simulink model "CrossCorrelation_SimulinkModel"  (R2018b)
settings: Solver=VariableStepAuto  StartTime=0.0  StopTime=0.1  RelTol=1e-3
libraries: dspstat3 x1
settings Model: Creator=Jayef  LastModifiedBy=Jayef

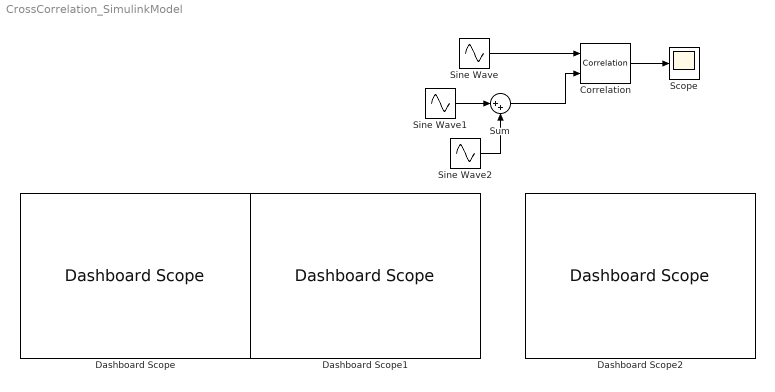
== system CrossCorrelation_SimulinkModel ==
  Correlation : dspstat3/Correlation  domain=Time  roundingMode=Floor  overflowMode=off  outputDataTypeStr=Inherit: Same as accumulator  outputMin=[]  outputMax=[]  outputLastDataTypeStr=Inherit: Same as accumulator
      settings: SourceProductName=DSP System Toolbox  SourceProductBaseCode=DS
  Dashboard Scope : DashboardScope  WebBlockId=4
  Dashboard Scope1 : DashboardScope  WebBlockId=9
  Dashboard Scope2 : DashboardScope  WebBlockId=10
  Scope : Scope
  Sine Wave : Sin  Frequency=2*3.14*50  SampleTime=1/1000
  Sine Wave1 : Sin  Frequency=2*3.14*50  SampleTime=1/1000
  Sine Wave2 : Sin  Amplitude=0.23  Frequency=2*3.14*70  SampleTime=1/1000
  Sum : Sum  Inputs=|++
  wires:
  Sine Wave/1 -> Correlation/1
  Sine Wave1/1 -> Sum/1
  Sine Wave2/1 -> Sum/2
  Sum/1 -> Correlation/2
  Correlation/1 -> Scope/1
